simulink library "Inverter"  (R2018b)
settings: Solver=ode45  StartTime=0.0  StopTime=10.0  RelTol=1e-3  EnableMultiTasking=on
undefined symbols (not defined in the file): ActPower1, ActPower2, ActPower3, Frequency, path_carnot, phase, Voltage1, Voltage2, Voltage3
libraries: simulink x1, carnot x1
settings Model: Creator=bernd.hafner  LastModifiedBy=drhf
settings DataIOCC: LimitDataPoints=on  SaveFormat=Array  SignalLoggingSaveFormat=ModelDataLogs
settings OptimizationCC: ExpressionDepthLimit=2147483647  LifeSpan=inf
settings DebuggingCC: UnderspecifiedInitializationDetection=Classic  MergeDetectMultiDrivingBlocksExec=none  SolverPrmCheckMsg=warning  FcnCallInpInsideContextMsg=warning  StateNameClashWarn=warning  SFUnexpectedBacktrackingDiag=warning  SFNoUnconditionalDefaultTransitionDiag=warning  SFExecutionAtInitializationDiag=none
settings HardwareCC: ProdBitPerPointer=32  ProdBitPerSizeT=32  ProdBitPerPtrDiffT=32  ProdLargestAtomicFloat=None  ProdIntDivRoundTo=Undefined  ProdEndianess=Unspecified  ProdWordSize=32  ProdHWDeviceType=32-bit Generic
settings ModelReferenceCC: PropagateSignalLabelsOutOfModel=off
settings SFSimCC: SimUseLocalCustomCode=off
settings RTWCC: RTWUseLocalCustomCode=off
settings CodeAppCC: StateflowObjectComments=on
settings GRTTargetCC: TargetLangStandard=C89/C90 (ANSI)  GeneratePreprocessorConditionals=Disable all  CombineOutputUpdateFcns=off  GRTInterface=on
settings ConfigComp: CovMetricSettings=dw  CovHtmlReporting=on  CovSaveCumulativeToWorkspaceVar=on  CovSaveSingleToWorkspaceVar=on  CovExternalEMLEnable=off

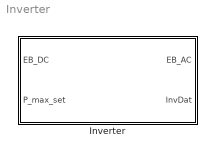
== system Inverter ==
  Inverter : Subsystem  mask(Inverter){PathName=fullfile(path_carnot('libsl'), 'Source', 'Electric_Generator', 'Inverter', 'parameter_set'), FileName='SMA_SB1_5_VL40.mat', userPath=off, userParam=off, Pacnom=1500, nphase=1-phase, U=230, f=50, PstepsEta=[0 0.1 0.2 0.25 0.3 0.5 0.75 1], Eta=[0 0.927 0.955 0.96 0.964 0.97 0.972 0.972], P_standby=1}
      mask prompts: PathName "Path"; FileName "Parameter set"; userPath "Edit path and name of parameter set"; userParam "User defined parameters"; Pacnom "Maximum AC power in W"; nphase "Number of phases"; U "Voltage of grid"; f "Frequency of grid"; PstepsEta "Breakpoints for efficiency (0..1)"; Eta "Efficiency table data (0..1)"; P_standby "Standby power in W"
      mask help: Model of an inverter e.g. for PV generators. The block considers the eficiency of the inverter in a lookup table.
      mask init:
      | % callback to set parameters of model
      | [ok, param] = CarnotCallbacks_InverterConf('SetParameters',gcbh,PathName,FileName);
      mask Help: web(fullfile(path_carnot('help'),'Inverter.html'),'-helpbrowser')
      mask Callback userPath: [ok, param] = CarnotCallbacks_InverterConf('UserEdit',gcbh);
      mask Callback userParam: [ok, param] = CarnotCallbacks_InverterConf('UserEdit',gcbh);
      mask TypeOptions Pacnom: NormialPower/Value | limit_Pacnom/UpperLimit
      mask TypeOptions nphase: Nphase/nphase
      mask TypeOptions U: Voltage/Value
      mask TypeOptions f: Frequency/Value
      mask TypeOptions PstepsEta: 1-D Lookup Table/BreakpointsForDimension1
      mask TypeOptions Eta: 1-D Lookup Table/Table
      mask TypeOptions P_standby: P_standby/Value
      mask DialogControl ParameterGroupFile Prompt: Picking a parameter set
      mask DialogControl Control2 Prompt: Carnot public data
      mask DialogControl Control2 Callback: [ok, file] = CarnotCallbacks_InverterConf('GetFilename',gcbh,'public');
      mask DialogControl Control3 Prompt: Carnot internal data
      mask DialogControl Control3 Callback: [ok, file] = CarnotCallbacks_InverterConf('GetFilename',gcbh,'internal');
      mask DialogControl Control4 Prompt: Selected path
      mask DialogControl Control4 Callback: [ok, file] = CarnotCallbacks_InverterConf('GetFilename',gcbh,'selected');
      mask DialogControl Control5 Prompt: Save in Carnot internal data
      mask DialogControl Control5 Callback: [ok, param] = CarnotCallbacks_InverterConf('SaveFilename',gcbh,'internal','IVRT');
      mask DialogControl Control6 Prompt: Save in selected path
      mask DialogControl Control6 Callback: [ok, param] = CarnotCallbacks_InverterConf('SaveFilename',gcbh,'selected','IVRT');
      mask Display:
      | pic = false;
      | if ~BlockIsInCarnotLibrary    % if not located in library any more
      |     picfile = fullfile(path_carnot('intlibsl'), ...
      |         'Source','Electric_Generator','Inverter','parameter_set', ...
      |         'Inverter.jpg');
      |     if exist(picfile,'file') % show internal picture if defined
      |         image(imread(picfile), [0.2, 0, 0.6, 1])
      |         set_param(gcb, 'BackgroundColor', 'White')
      |         pic = true;
      |     end
      | end
      | if ~pic    % show public picture
      |     set_param(gcb, 'BackgroundColor', 'Orange')
      |     plot(-40,0,140,100,...
      |         [90,10,90,90,10,10],[10,90,90,10,10,90],...
      |         [40,20],[40,40],[40,20],[30,30],...
      |         [88,84,75,64,55,50],[70,60,60,80,80,70])
      | end

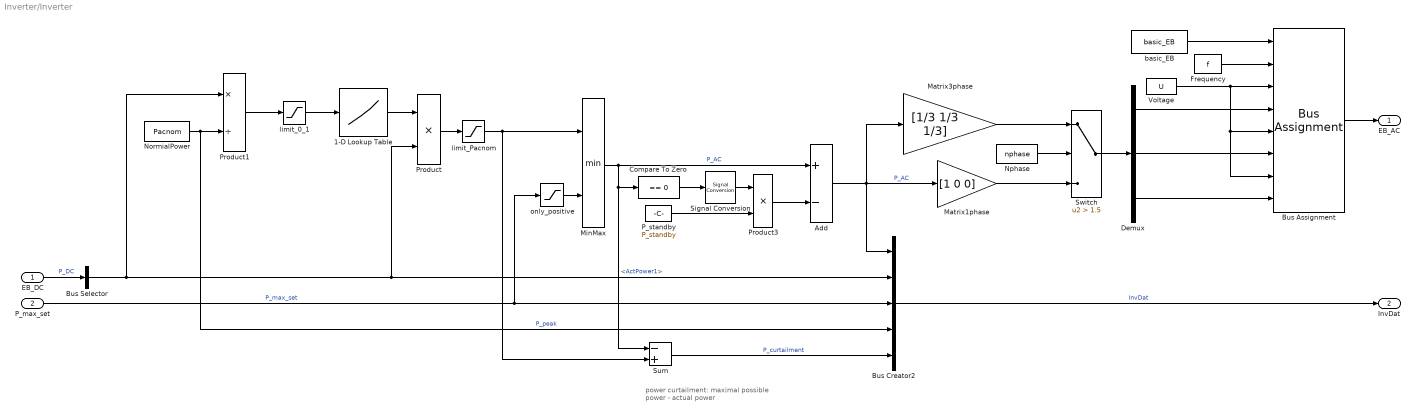
== system Inverter/Inverter ==
  note: power curtailment:
      | maximal possible power - actual power
  EB_DC : Inport
  P_max_set : Inport  Port=2
  1-D Lookup Table : Lookup_n-D  NumberOfTableDimensions=1  BreakpointsForDimension1=PstepsEta  Table=Eta  RndMeth=Simplest  InputSameDT=on
  Add : Sum  Inputs=+-
  Bus Assignment : BusAssignment  AssignedSignals=Frequency,Voltage1,ActPower1,Voltage2,ActPower2,Voltage3,ActPower3
  Bus Creator2 : BusCreator  Inputs=5
  Bus Selector : BusSelector  OutputSignals=ActPower1
  Compare To Zero : simulink/Logic and Bit Operations/Compare To Zero  relop===  OutDataTypeStr=boolean
  Demux : Demux  Outputs=3
  Frequency : Constant  Value=f
  Matrix1phase : Gain  Gain=[1 0 0]
  Matrix3phase : Gain  Gain=[1/3 1/3 1/3]
  MinMax : MinMax  Inputs=2
  NormialPower : Constant  Value=Pacnom
  Nphase : Constant  Value=nphase  mask{nphase=1-phase}
      mask prompts: nphase "Number of phases"
      mask TypeOptions nphase: 1-phase | 3-phase
  P_standby : Constant  Value=P_standby
  Product : Product
  Product1 : Product  Inputs=*/
  Product3 : Product
  Signal Conversion : SignalConversion  OverrideOpt=off
  Sum : Sum  Inputs=-+
  Switch : Switch  Criteria=u2 > Threshold  Threshold=1.5
  Voltage : Constant  Value=U
  basic_EB : carnot/Basic/Electric/basic_EB  eID=Power only  f=50  v1=230  p1=0  pf1=1  v2=230  p2=0  pf2=1  v3=230  p3=0  pf3=1
      settings: SourceProductName=Carnot
  limit_0_1 : Saturate  UpperLimit=inf  LowerLimit=0
  limit_Pacnom : Saturate  UpperLimit=Pacnom  LowerLimit=0
  only_positive : Saturate  UpperLimit=inf  LowerLimit=0
  EB_AC : Outport
  InvDat : Outport  Port=2
  wires:
  Bus Selector/1 -> Product1/1, Bus Creator2/2, Product/2  "<ActPower1>"
  EB_DC/1 -> Bus Selector/1  "P_DC"
  P_max_set/1 -> only_positive/1, Bus Creator2/3  "P_max_set"
  MinMax/1 -> Add/1, Compare To Zero/1, Sum/1  "P_AC"
  Bus Creator2/1 -> InvDat/1  "InvDat"
  Sum/1 -> Bus Creator2/5  "P_curtailment"
  Product1/1 -> limit_0_1/1
  NormialPower/1 -> Bus Creator2/4, Product1/2  "P_peak"
  only_positive/1 -> MinMax/2
  Product/1 -> limit_Pacnom/1
  1-D Lookup Table/1 -> Product/1
  Compare To Zero/1 -> Signal Conversion/1
  Signal Conversion/1 -> Product3/1
  P_standby/1 -> Product3/2
  Product3/1 -> Add/2
  Add/1 -> Matrix3phase/1, Matrix1phase/1, Bus Creator2/1  "P_AC"
  basic_EB/1 -> Bus Assignment/1
  Bus Assignment/1 -> EB_AC/1
  Frequency/1 -> Bus Assignment/2
  Voltage/1 -> Bus Assignment/7, Bus Assignment/5, Bus Assignment/3
  Demux/2 -> Bus Assignment/6
  Demux/3 -> Bus Assignment/8
  Demux/1 -> Bus Assignment/4
  Switch/1 -> Demux/1
  Matrix1phase/1 -> Switch/3
  Matrix3phase/1 -> Switch/1
  Nphase/1 -> Switch/2
  limit_0_1/1 -> 1-D Lookup Table/1
  limit_Pacnom/1 -> Sum/2, MinMax/1
